simulink model "lab2_model_ssEmulation_choices"  (R2024b)
settings: Solver=FixedStepAuto  StartTime=0.0  StopTime=sIn.simulation_time  FixedStep=sIn.step_size
values from neighbouring files (symbols this model uses):
  obsD = obs.tmp(sIn.integrationMethod)    [lab2_startup_ssEmulation.m]
undefined symbols (not defined in the file or in its folder): DiscIntNeverNeededParam, drv, feedback, gbox, mld, mot, rads2rpm, rpm2rads, sens, sIn
libraries: simulink_extras x1, simulink x1
settings Model: Creator=bmm1  LastModifiedBy=pries
settings RTWCC: GPUComputeCapability=3.5

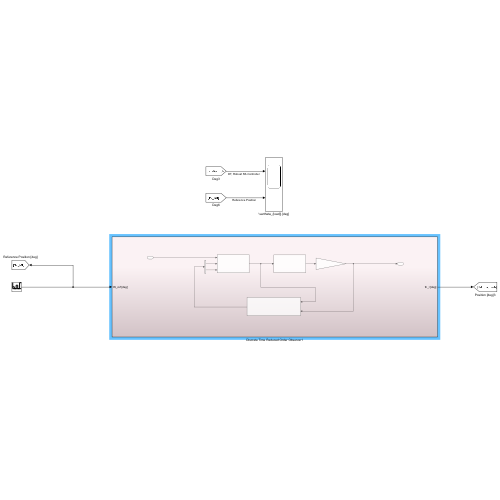
[thumbnail: Simulink's stored preview of the top-level diagram]
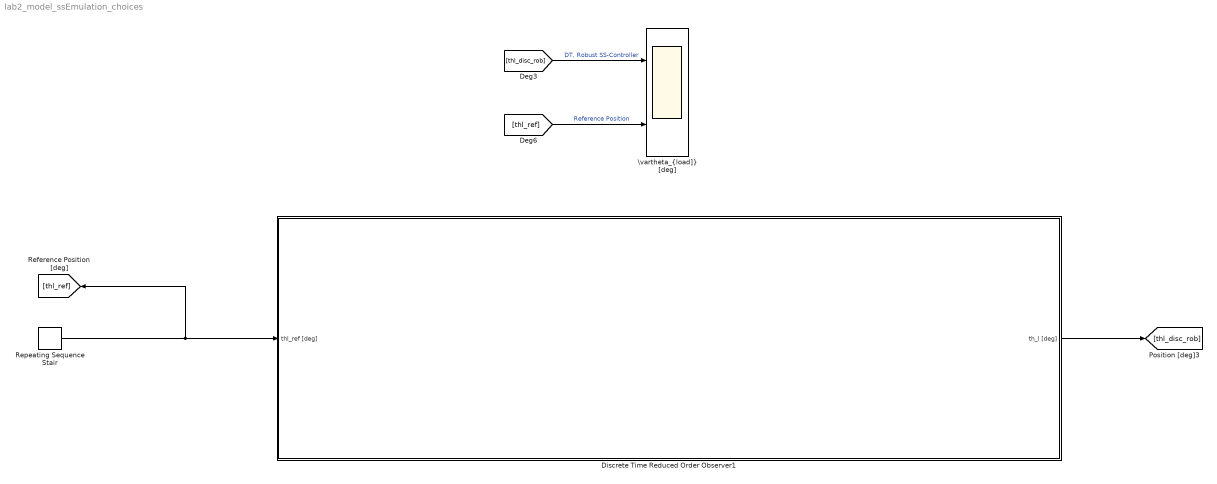
== system lab2_model_ssEmulation_choices ==
  Discrete Time Reduced Order Observer1 : Subsystem
  Repeating Sequence Stair : simulink/Sources/Repeating Sequence Stair  OutValues=sIn.position  tsamp=sIn.sample_time  OutMin=[]  OutMax=[]  OutDataTypeStr=double  OutputDataTypeScalingMode=double  OutDataType=fixdt(0,8)  ConRadixGroup=Best Precision: Vector-wise  OutScaling=2^-12
  "\\vartheta_{load]} [deg]" : Scope  NumInputPorts=2
  wires:
  [thl_ref] -> "\\vartheta_{load]} [deg]"/2  "Reference Position"
  Repeating Sequence Stair/1 -> Discrete Time Reduced Order Observer1/1(thl_ref [deg]), [thl_ref]
  Discrete Time Reduced Order Observer1/1(th_l [deg]) -> [thl_disc_rob]
  [thl_disc_rob] -> "\\vartheta_{load]} [deg]"/1  "DT, Robust SS-Controller"

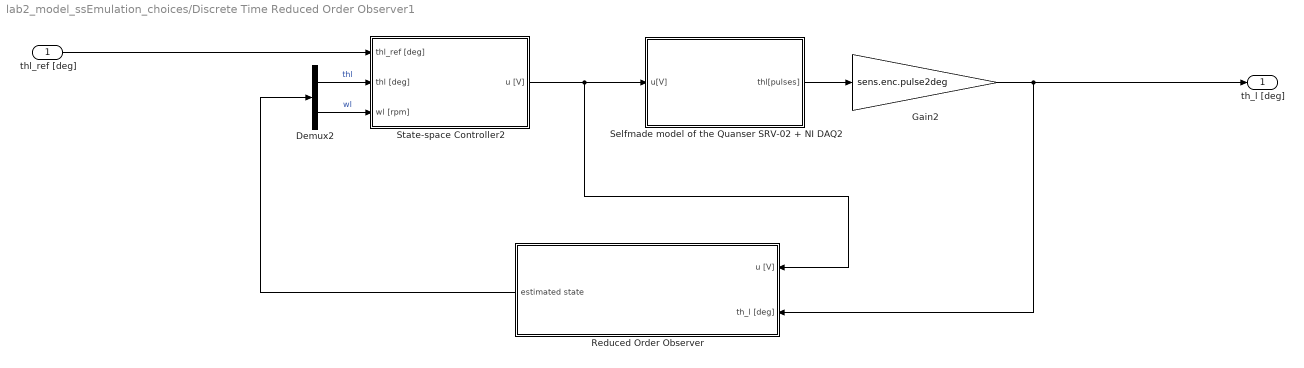
== system lab2_model_ssEmulation_choices/Discrete Time Reduced Order Observer1 ==
  thl_ref [deg] : Inport
  Demux2 : Demux  Outputs=2
  Gain2 : Gain  Gain=sens.enc.pulse2deg
  Reduced Order Observer : Subsystem
  Selfmade model of the Quanser SRV-02 + NI DAQ2 : Subsystem
  State-space Controller2 : Subsystem
  th_l [deg] : Outport
  wires:
  thl_ref [deg]/1 -> State-space Controller2/1(thl_ref [deg])
  Demux2/1 -> State-space Controller2/2(thl [deg])  "thl"
  Demux2/2 -> State-space Controller2/3(wl [rpm])  "wl"
  Selfmade model of the Quanser SRV-02 + NI DAQ2/1(thl[pulses]) -> Gain2/1
  Gain2/1 -> Reduced Order Observer/2(th_l [deg]), th_l [deg]/1
  State-space Controller2/1(u [V]) -> Reduced Order Observer/1(u [V]), Selfmade model of the Quanser SRV-02 + NI DAQ2/1(u[V])
  Reduced Order Observer/1(estimated state) -> Demux2/1

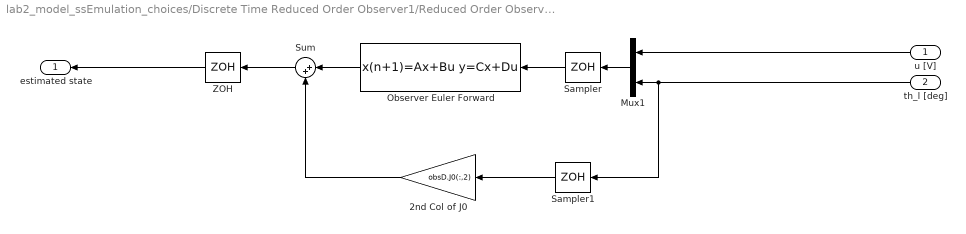
== system lab2_model_ssEmulation_choices/Discrete Time Reduced Order Observer1/Reduced Order Observer ==
  u [V] : Inport
  th_l [deg] : Inport  Port=2
  2nd Col of J0 : Gain  Gain=obsD.J0(:,2)
  Mux1 : Mux  Inputs=2
  Observer Euler Forward : DiscreteStateSpace  A=obsD.Phi0  B=obsD.Gamma0  C=obsD.H0  D=zeros(2,2)  SampleTime=sIn.Ts
  Sampler : ZeroOrderHold  SampleTime=sIn.Ts
  Sampler1 : ZeroOrderHold  SampleTime=sIn.Ts
  Sum : Sum  Inputs=|++
  ZOH : ZeroOrderHold  SampleTime=sIn.Ts
  estimated state : Outport
  wires:
  Sampler/1 -> Observer Euler Forward/1
  Sum/1 -> ZOH/1
  Observer Euler Forward/1 -> Sum/1
  Sampler1/1 -> 2nd Col of J0/1
  Mux1/1 -> Sampler/1
  2nd Col of J0/1 -> Sum/2
  th_l [deg]/1 -> Sampler1/1, Mux1/2
  u [V]/1 -> Mux1/1
  ZOH/1 -> estimated state/1

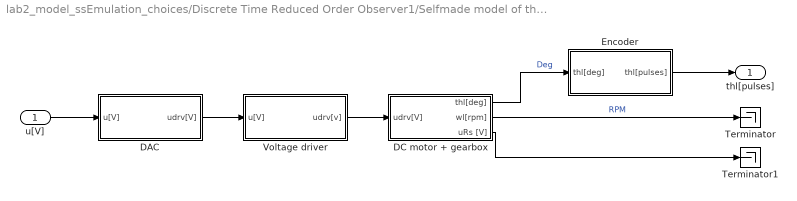
== system lab2_model_ssEmulation_choices/Discrete Time Reduced Order Observer1/Selfmade model of the Quanser SRV-02 + NI DAQ2 ==
  u[V] : Inport
  DAC : Subsystem
  DC motor + gearbox : Subsystem
  Encoder : Subsystem
  Terminator : Terminator
  Terminator1 : Terminator
  Voltage driver : Subsystem
  thl[pulses] : Outport
  wires:
  DC motor + gearbox/1(thl[deg]) -> Encoder/1(thl[deg])  "Deg"
  u[V]/1 -> DAC/1(u[V])
  DC motor + gearbox/2(wl[rpm]) -> Terminator/1  "RPM"
  DAC/1(udrv[V]) -> Voltage driver/1(u[V])
  Voltage driver/1(udrv[v]) -> DC motor + gearbox/1(udrv[V])
  Encoder/1(thl[pulses]) -> thl[pulses]/1
  DC motor + gearbox/3(uRs [V]) -> Terminator1/1

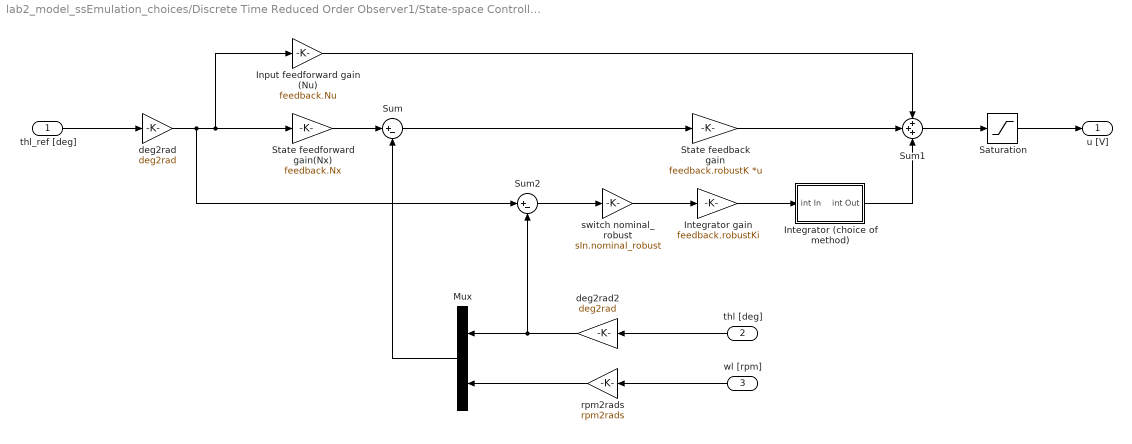
== system lab2_model_ssEmulation_choices/Discrete Time Reduced Order Observer1/State-space Controller2 ==
  thl_ref [deg] : Inport
  thl [deg] : Inport  Port=2
  wl [rpm] : Inport  Port=3
  Input feedforward gain (Nu) : Gain  Gain=feedback.Nu
  Integrator (choice of method) : Subsystem
  Integrator gain : Gain  Gain=feedback.robustKi
  Mux : Mux  Inputs=2
  Saturation : Saturate  UpperLimit=10  LowerLimit=-10
  State feedback gain : Gain  Gain=feedback.robustK  Multiplication=Matrix(K*u)
  State feedforward gain(Nx) : Gain  Gain=feedback.Nx
  Sum : Sum  Inputs=|+-
  Sum1 : Sum  Inputs=+++
  Sum2 : Sum  Inputs=|+-
  deg2rad : Gain  Gain=deg2rad
  deg2rad2 : Gain  Gain=deg2rad
  rpm2rads : Gain  Gain=rpm2rads
  switch nominal_robust : Gain  Gain=sIn.nominal_robust
  u [V] : Outport
  wires:
  thl_ref [deg]/1 -> deg2rad/1
  deg2rad/1 -> Sum2/1, Input feedforward gain (Nu)/1, State feedforward gain(Nx)/1
  State feedforward gain(Nx)/1 -> Sum/1
  Sum/1 -> State feedback gain/1
  State feedback gain/1 -> Sum1/2
  Input feedforward gain (Nu)/1 -> Sum1/1
  Sum1/1 -> Saturation/1
  Saturation/1 -> u [V]/1
  thl [deg]/1 -> deg2rad2/1
  wl [rpm]/1 -> rpm2rads/1
  deg2rad2/1 -> Sum2/2, Mux/1
  rpm2rads/1 -> Mux/2
  Mux/1 -> Sum/2
  Sum2/1 -> switch nominal_robust/1
  Integrator gain/1 -> Integrator (choice of method)/1(int In)
  Integrator (choice of method)/1(int Out) -> Sum1/3
  switch nominal_robust/1 -> Integrator gain/1

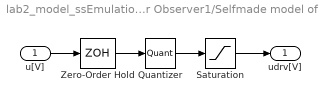
== system lab2_model_ssEmulation_choices/Discrete Time Reduced Order Observer1/Selfmade model of the Quanser SRV-02 + NI DAQ2/DAC ==
  u[V] : Inport
  Quantizer : Quantizer  QuantizationInterval=daq.dac.q
  Saturation : Saturate  UpperLimit=10  LowerLimit=-10
  Zero-Order Hold : ZeroOrderHold  SampleTime=1e-3
  udrv[V] : Outport
  wires:
  Zero-Order Hold/1 -> Quantizer/1
  u[V]/1 -> Zero-Order Hold/1
  Quantizer/1 -> Saturation/1
  Saturation/1 -> udrv[V]/1

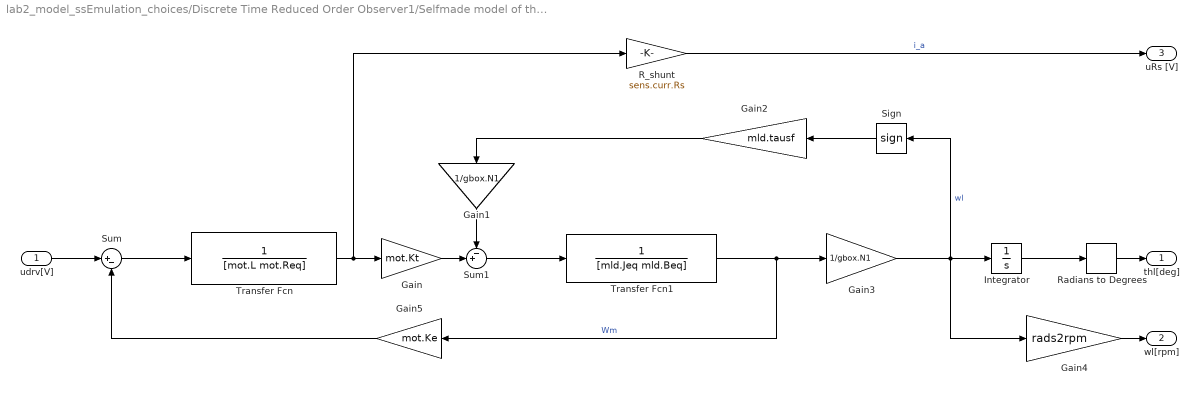
== system lab2_model_ssEmulation_choices/Discrete Time Reduced Order Observer1/Selfmade model of the Quanser SRV-02 + NI DAQ2/DC motor + gearbox ==
  udrv[V] : Inport
  Gain : Gain  Gain=mot.Kt
  Gain1 : Gain  Gain=1/gbox.N1
  Gain2 : Gain  Gain=mld.tausf
  Gain3 : Gain  Gain=1/gbox.N1
  Gain4 : Gain  Gain=rads2rpm
  Gain5 : Gain  Gain=mot.Ke
  Integrator : Integrator
  R_shunt : Gain  Gain=sens.curr.Rs
  Radians to Degrees : simulink_extras/Transformations/Radians to Degrees
  Sign : Signum  ZeroCross=off
  Sum : Sum  Inputs=|+-
  Sum1 : Sum  Inputs=-+|
  Transfer Fcn : TransferFcn  Denominator=[mot.L mot.Req]
  Transfer Fcn1 : TransferFcn  Denominator=[mld.Jeq mld.Beq]
  thl[deg] : Outport
  wl[rpm] : Outport  Port=2
  uRs [V] : Outport  Port=3
  wires:
  udrv[V]/1 -> Sum/1
  Sum/1 -> Transfer Fcn/1
  Transfer Fcn/1 -> R_shunt/1, Gain/1
  Gain1/1 -> Sum1/1
  Gain2/1 -> Gain1/1
  Sign/1 -> Gain2/1
  Transfer Fcn1/1 -> Gain5/1, Gain3/1  "Wm"
  Gain3/1 -> Gain4/1, Sign/1, Integrator/1  "wl"
  Integrator/1 -> Radians to Degrees/1
  Radians to Degrees/1 -> thl[deg]/1
  Gain4/1 -> wl[rpm]/1
  Sum1/1 -> Transfer Fcn1/1
  Gain/1 -> Sum1/2
  Gain5/1 -> Sum/2
  R_shunt/1 -> uRs [V]/1  "i_a"

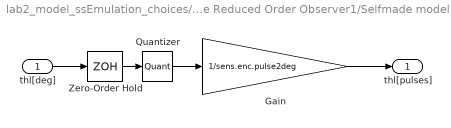
== system lab2_model_ssEmulation_choices/Discrete Time Reduced Order Observer1/Selfmade model of the Quanser SRV-02 + NI DAQ2/Encoder ==
  thl[deg] : Inport
  Gain : Gain  Gain=1/sens.enc.pulse2deg
  Quantizer : Quantizer  QuantizationInterval=sens.enc.pulse2deg
  Zero-Order Hold : ZeroOrderHold  SampleTime=1e-3
  thl[pulses] : Outport
  wires:
  thl[deg]/1 -> Zero-Order Hold/1
  Gain/1 -> thl[pulses]/1
  Quantizer/1 -> Gain/1
  Zero-Order Hold/1 -> Quantizer/1

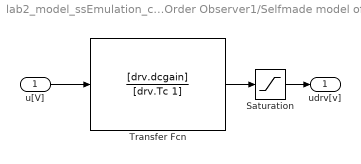
== system lab2_model_ssEmulation_choices/Discrete Time Reduced Order Observer1/Selfmade model of the Quanser SRV-02 + NI DAQ2/Voltage driver ==
  u[V] : Inport
  Saturation : Saturate  UpperLimit=12  LowerLimit=-12
  Transfer Fcn : TransferFcn  Numerator=[drv.dcgain]  Denominator=[drv.Tc 1]
  udrv[v] : Outport
  wires:
  u[V]/1 -> Transfer Fcn/1
  Transfer Fcn/1 -> Saturation/1
  Saturation/1 -> udrv[v]/1

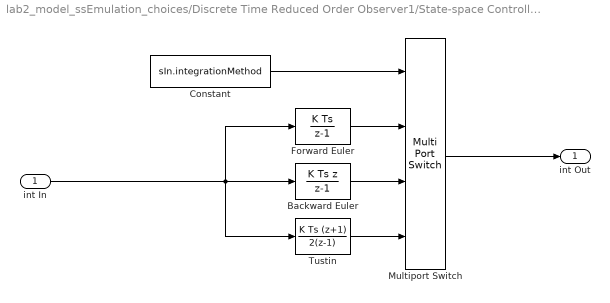
== system lab2_model_ssEmulation_choices/Discrete Time Reduced Order Observer1/State-space Controller2/Integrator (choice of method) ==
  int In : Inport
  Backward Euler : DiscreteIntegrator  IntegratorMethod=Integration: Backward Euler  SampleTime=sIn.Ts  ICPrevOutput=DiscIntNeverNeededParam  ICPrevScaledInput=DiscIntNeverNeededParam
  Constant : Constant  Value=sIn.integrationMethod
  Forward Euler : DiscreteIntegrator  SampleTime=sIn.Ts  ICPrevOutput=DiscIntNeverNeededParam  ICPrevScaledInput=DiscIntNeverNeededParam
  Multiport Switch : MultiPortSwitch  SaturateOnIntegerOverflow=off  InputSameDT=off
  Tustin : DiscreteIntegrator  IntegratorMethod=Integration: Trapezoidal  SampleTime=sIn.Ts  ICPrevOutput=DiscIntNeverNeededParam  ICPrevScaledInput=DiscIntNeverNeededParam
  int Out : Outport
  wires:
  Forward Euler/1 -> Multiport Switch/2
  Backward Euler/1 -> Multiport Switch/3
  Tustin/1 -> Multiport Switch/4
  int In/1 -> Tustin/1, Forward Euler/1, Backward Euler/1
  Constant/1 -> Multiport Switch/1
  Multiport Switch/1 -> int Out/1
